simulink model "simGenerateData"  (R2015b)
settings: Solver=VariableStepAuto  StartTime=0.0  StopTime=totalTime  RelTol=1e-3
values from neighbouring files (symbols this model uses):
  cVal = c(lN)    [generateData.m]
  eVal = e(kN)    [generateData.m]
  lVal = l(jN)    [generateData.m]
  rVal = r(iN)    [generateData.m]
  t1 = normrnd(tStartMean, tStartSD)    [generateData.m]
  t2 = normrnd(tStopMean, tStopSD)    [generateData.m]
  totalTime = 25e-6    (= 2.5e-05)    [generateData.m]
  vVal = v(mN)    [generateData.m]
libraries: powerlib x9
settings Model: Creator=akshay  LastModifiedBy=akshay

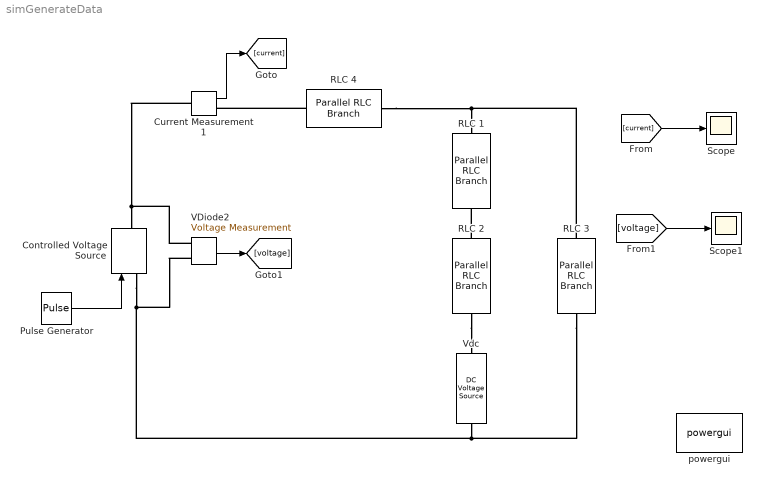
== system simGenerateData ==
  " RLC 1" : powerlib/Elements/Parallel RLC Branch  LConnTagsString=a  RConnTagsString=__new0  BranchType=R  Resistance=rVal  Inductance=1e-3  SetiL0=off  InitialCurrent=0  Capacitance=0.1e-6  Setx0=off  InitialVoltage=0  Measurements=None
  " RLC 2" : powerlib/Elements/Parallel RLC Branch  LConnTagsString=a  RConnTagsString=__new0  BranchType=L  Resistance=rVal  Inductance=lVal  SetiL0=off  InitialCurrent=0  Capacitance=0.1e-6  Setx0=off  InitialVoltage=0  Measurements=None
  " RLC 3" : powerlib/Elements/Parallel RLC Branch  LConnTagsString=a  RConnTagsString=__new0  BranchType=C  Resistance=rVal  Inductance=1e-3  SetiL0=off  InitialCurrent=0  Capacitance=cVal  Setx0=off  InitialVoltage=0  Measurements=None
  " RLC 4" : powerlib/Elements/Parallel RLC Branch  LConnTagsString=a  RConnTagsString=__new0  BranchType=R  Resistance=0.001  Inductance=1e-3  SetiL0=off  InitialCurrent=0  Capacitance=0.1e-6  Setx0=off  InitialVoltage=0  Measurements=None
  Controlled Voltage Source : powerlib/Electrical Sources/Controlled Voltage Source  Initialize=on  Source_Type=AC  Amplitude=0  Phase=0  Frequency=0  Measurements=None
  Current Measurement1 : powerlib/Measurements/Current Measurement  PhasorSimulation=off  OutputType=Complex  PSBequivalent=0
  Pulse Generator : DiscretePulseGenerator  PulseType=Time based  Amplitude=vVal  Period=totalTime  PulseWidth=100*(t2-t1)/totalTime  PhaseDelay=t1
  Scope : Scope
  Scope1 : Scope
  VDiode2 : powerlib/Measurements/Voltage Measurement  PhasorSimulation=off  OutputType=Complex  PSBequivalent=0
  Vdc : powerlib/Electrical Sources/DC Voltage Source  Amplitude=eVal  Measurements=Voltage
  powergui : powerlib/powergui  Priority=1  SimulationMode=Continuous  SolverType=Tustin/Backward Euler (TBE)  SampleTime=50e-6  frequency=60  SPID=off  DisableSnubberDevices=off  DisableRonSwitches=off  DisableVfSwitches=off  SwTol=0  DisplayEquations=off  Interpol=off  ExternalGateDelay=off  methode=off  Ts=10  FunctionMessages=off  echomessages=off  HookPort=off  EnableUseOfTLC=off  x0status=blocks  frequencyindice=0  Pbase=100e6  ErrMax=1e-4  Iterations=50  UnitsV=kV  UnitsW=MW  buscounter=0  RestoreLinks=warning  ResistiveCurrentMeasurement=off  Frange=[0:2:500]  Ylog=off  Xlog=on  ShowGrid=off  save=off  variable=ZData  structure=0  ZoomFFT=off  StartTime=0.0  cycles=1  DisplayStyle=1  fundamental=60  FreqAxis=off  MaxFrequency=1000  frequencyindicesteady=1  RmsSteady=1  display=off
  wires:
  Pulse Generator/1 -> Controlled Voltage Source/1
  Current Measurement1/1 -> [current]
  VDiode2/1 -> [voltage]
  [current] -> Scope/1
  [voltage] -> Scope1/1
  connections:
  Current Measurement1/LConn1 -- VDiode2/LConn1 -- Controlled Voltage Source/RConn1
  Vdc/LConn1 -- " RLC 3"/RConn1 -- Controlled Voltage Source/LConn1 -- VDiode2/LConn2
  " RLC 2"/LConn1 -- " RLC 1"/RConn1
  " RLC 2"/RConn1 -- Vdc/RConn1
  " RLC 4"/RConn1 -- Current Measurement1/RConn1
  " RLC 4"/LConn1 -- " RLC 1"/LConn1 -- " RLC 3"/LConn1
